simulink model "regulator_2"  (R2016a)
settings: Solver=VariableStepAuto  SolverMode=SingleTasking  StartTime=0.0  StopTime=tfinal  RelTol=1e-3
values from neighbouring files (symbols this model uses):
  AA = A    [identify_v2.m]    (also in statespace.mat = [5.5279791139 1 0 0 0 0 0 -13.5203927489 0 1 0 0 ... (49 ele)
  BB = B    [identify_v2.m]    (also in statespace.mat = [1 0 0 0 0 0 0])
  CC = C    [identify_v2.m]    (also in statespace.mat = [-3.36334453848e-05 3.71652773519e-05 -0.000281908447517 0.0)
  Nbar = Nu+K*Nx    [controller.m]
  Ts = mean(diff(ts))    [controller.m]    (also in identify.m; identify_v2.m; simubarra1.m = 0.01)
undefined symbols (not defined in the file or in its folder): K, M
settings Model: Creator=Pedro Palmeiro  LastModifiedBy=Pedro Palmeiro
settings DataIOCC: ReturnWorkspaceOutputs=on
settings DebuggingCC: SFUnexpectedBacktrackingDiag=error  SFNoUnconditionalDefaultTransitionDiag=error
settings SFSimCC: SimUseLocalCustomCode=on
settings RTWCC: RTWUseLocalCustomCode=on
settings GRTTargetCC: TargetLangStandard=C99 (ISO)  GeneratePreprocessorConditionals=Use local settings
settings ConfigComp: CovMetricSettings=dwe  CovHtmlReporting=off  CovSaveCumulativeToWorkspaceVar=off  CovSaveSingleToWorkspaceVar=off  CovExternalEMLEnable=on

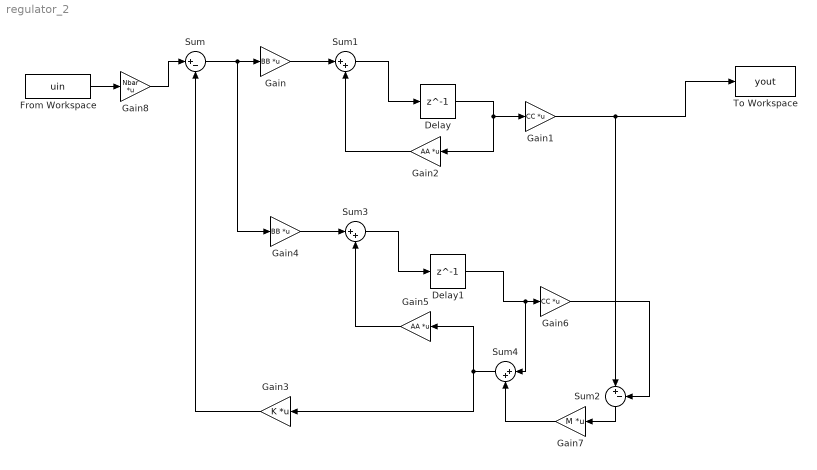
== system regulator_2 ==
  Delay : Delay  DelayLength=1  InitialCondition=0
  Delay1 : Delay  DelayLength=1  InitialCondition=0
  From Workspace : FromWorkspace  VariableName=uin  SampleTime=Ts
  Gain : Gain  Gain=BB  Multiplication=Matrix(K*u)
  Gain1 : Gain  Gain=CC  Multiplication=Matrix(K*u)
  Gain2 : Gain  Gain=AA  Multiplication=Matrix(K*u)
  Gain3 : Gain  Gain=K  Multiplication=Matrix(K*u)
  Gain4 : Gain  Gain=BB  Multiplication=Matrix(K*u)
  Gain5 : Gain  Gain=AA  Multiplication=Matrix(K*u)
  Gain6 : Gain  Gain=CC  Multiplication=Matrix(K*u)
  Gain7 : Gain  Gain=M  Multiplication=Matrix(K*u)
  Gain8 : Gain  Gain=Nbar  Multiplication=Matrix(K*u)
  Sum : Sum  Inputs=|+-
  Sum1 : Sum  Inputs=|++
  Sum2 : Sum  Inputs=|+-
  Sum3 : Sum  Inputs=|++
  Sum4 : Sum  Inputs=|++
  To Workspace : ToWorkspace  VariableName=yout  SaveFormat=Structure With Time  SampleTime=-1
  wires:
  Sum/1 -> Gain/1, Gain4/1
  Gain2/1 -> Sum1/2
  Delay/1 -> Gain1/1, Gain2/1
  Gain1/1 -> To Workspace/1, Sum2/1
  Sum1/1 -> Delay/1
  Gain/1 -> Sum1/1
  Gain3/1 -> Sum/2
  Gain4/1 -> Sum3/1
  Sum3/1 -> Delay1/1
  Gain5/1 -> Sum3/2
  Gain6/1 -> Sum2/2
  Sum2/1 -> Gain7/1
  Delay1/1 -> Sum4/1, Gain6/1
  Sum4/1 -> Gain3/1, Gain5/1
  Gain7/1 -> Sum4/2
  From Workspace/1 -> Gain8/1
  Gain8/1 -> Sum/1
